simulink model "elec3200lab3"  (R2016a)
settings: Solver=VariableStepAuto  StartTime=0.0  StopTime=10  RelTol=1e-3
settings Model: Creator=古乔  LastModifiedBy=古乔

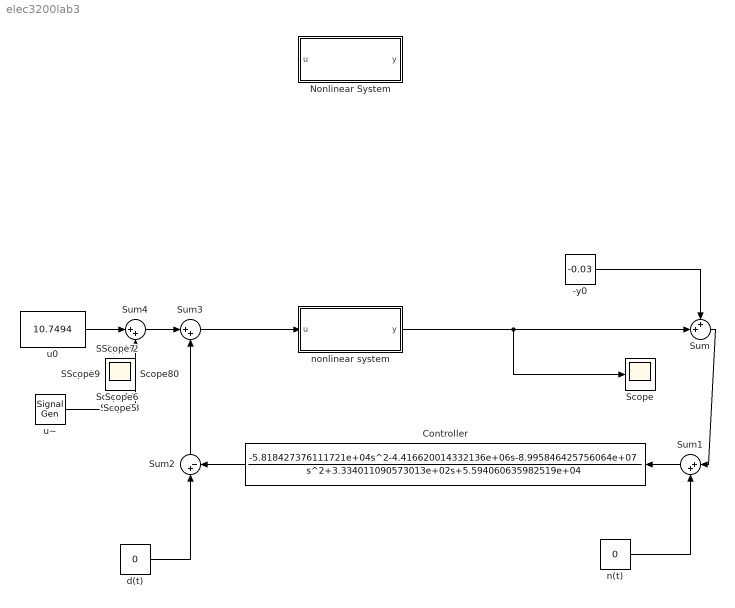
== system elec3200lab3 ==
  -y0 : Constant  Value=-0.03
  Controller : TransferFcn  Numerator=[-5.818427376111721e+04 -4.416620014332136e+06 -8.995846425756064e+07]  Denominator=[1 3.334011090573013e+02 5.594060635982519e+04]
  Nonlinear System : Subsystem
  Scope{,1..14} (15 alike) : Scope
  Sum : Sum  Inputs=++|
  Sum1 : Sum  Inputs=|++
  Sum2 : Sum  Inputs=|+-
  Sum3 : Sum  Inputs=|++
  Sum4 : Sum  Inputs=|++
  "d(t) " : Constant  Value=0
  "n(t) " : Constant  Value=0
  nonlinear system : Subsystem
  u0 : Constant  Value=10.7494
  u~ : SignalGenerator  WaveForm=square  Units=rad/sec
  wires:
  -y0/1 -> Sum/1
  Sum/1 -> Sum1/1
  Sum1/1 -> Controller/1
  "n(t) "/1 -> Sum1/2
  Controller/1 -> Sum2/2
  "d(t) "/1 -> Sum2/1
  Sum2/1 -> Sum3/2
  u0/1 -> Sum4/1
  Sum3/1 -> nonlinear system/1(u)
  nonlinear system/1(y) -> Sum/2, Scope/1
  Sum4/1 -> Sum3/1
  u~/1 -> Sum4/2

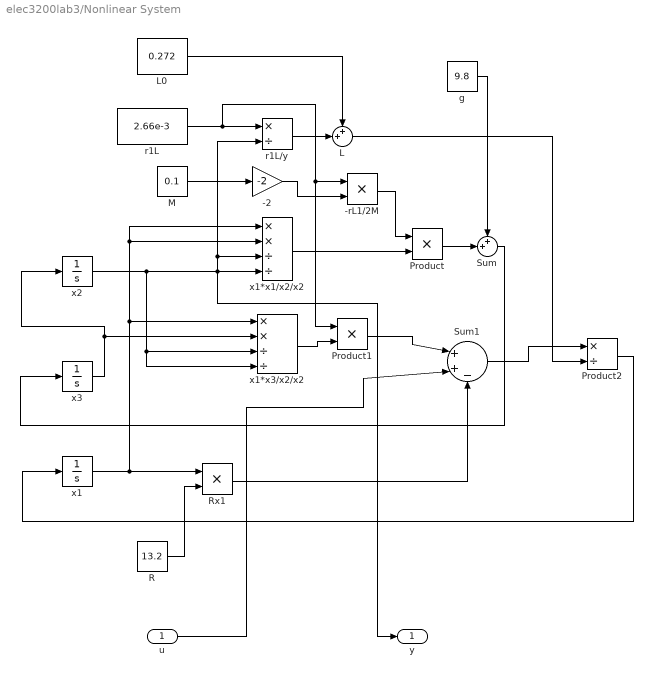
== system elec3200lab3/Nonlinear System ==
  u : Inport
  -2 : Gain  Gain=-2
  -rL1/2M : Product
  L : Sum  Inputs=++|
  L0 : Constant  Value=0.272
  M : Constant  Value=0.1
  Product : Product
  Product1 : Product
  Product2 : Product  Inputs=*/
  R : Constant  Value=13.2
  Rx1 : Product
  Sum : Sum  Inputs=++|
  Sum1 : Sum  Inputs=|++-
  g : Constant  Value=9.8
  r1L : Constant  Value=2.66e-3
  r1L/y : Product  Inputs=*/
  x1 : Integrator  InitialCondition=0.8143
  x1*x1/x2/x2 : Product  Inputs=**//
  x1*x3/x2/x2 : Product  Inputs=**//
  x2 : Integrator  InitialCondition=0.0300
  x3 : Integrator
  y : Outport
  wires:
  x1/1 -> Rx1/1, x1*x1/x2/x2/1, x1*x1/x2/x2/2, x1*x3/x2/x2/1
  x2/1 -> y/1, r1L/y/2, x1*x1/x2/x2/3, x1*x1/x2/x2/4, x1*x3/x2/x2/4, x1*x3/x2/x2/3
  r1L/1 -> Product1/1, -rL1/2M/1, r1L/y/1
  r1L/y/1 -> L/2
  L0/1 -> L/1
  L/1 -> Product2/2
  x3/1 -> x2/1, x1*x3/x2/x2/2
  M/1 -> -2/1
  -2/1 -> -rL1/2M/2
  -rL1/2M/1 -> Product/1
  x1*x1/x2/x2/1 -> Product/2
  Product/1 -> Sum/2
  g/1 -> Sum/1
  Sum/1 -> x3/1
  x1*x3/x2/x2/1 -> Product1/2
  R/1 -> Rx1/2
  u/1 -> Sum1/2
  Product1/1 -> Sum1/1
  Rx1/1 -> Sum1/3
  Sum1/1 -> Product2/1
  Product2/1 -> x1/1

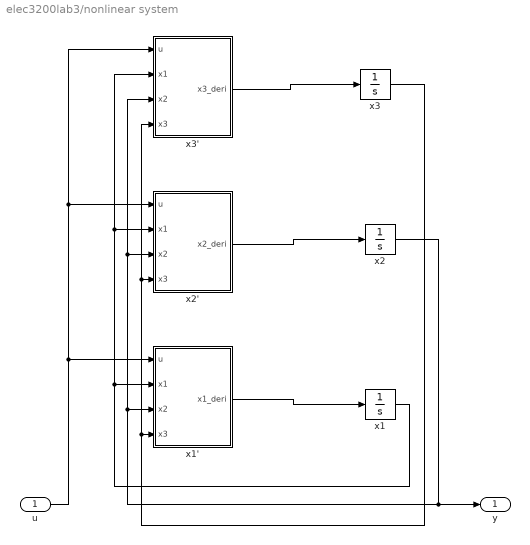
== system elec3200lab3/nonlinear system ==
  u : Inport
  x1 : Integrator  InitialCondition=0.84
  x1' : MATLAB Function  TreatAsAtomicUnit=on
  x2 : Integrator  InitialCondition=0.03
  x2' : MATLAB Function  TreatAsAtomicUnit=on
  x3 : Integrator
  x3' : MATLAB Function  TreatAsAtomicUnit=on
  y : Outport
  wires:
  u/1 -> x3'/1(u), x2'/1(u), x1'/1(u)
  x1'/1(x1_deri) -> x1/1
  x2'/1(x2_deri) -> x2/1
  x3'/1(x3_deri) -> x3/1
  x3/1 -> x3'/4(x3), x2'/4(x3), x1'/4(x3)
  x2/1 -> y/1, x3'/3(x2), x2'/3(x2), x1'/3(x2)
  x1/1 -> x1'/2(x1), x2'/2(x1), x3'/2(x1)

== matlab function elec3200lab3/nonlinear system/x2' ==
  data: u input; x1 input; x2_deri output; x2 input; x3 input
function x2_deri  = cal_dx2(u,x1,x2,x3)
y0 = 0.03;
L0 = 0.272;
R = 13.2;
M = 0.1;
rL1 = 2.66e-3;
g = 9.8;
L = L0 + rL1/x2;

x2_deri = x3;

== matlab function elec3200lab3/nonlinear system/x1' ==
  data: u input; x1 input; x1_deri output; x2 input; x3 input
function x1_deri  = cal_dx1(u,x1,x2,x3)
y0 = 0.03;
L0 = 0.272;
R = 13.2;
M = 0.1;
rL1 = 2.66e-3;
g = 9.8;
L = L0 + rL1/x2;

x1_deri = (u-R*x1+rL1*x1*x3/x2/x2)/L;

== matlab function elec3200lab3/nonlinear system/x3' ==
  data: u input; x1 input; x3_deri output; x2 input; x3 input
function x3_deri  = cal_dx3(u,x1,x2,x3)
y0 = 0.03;
L0 = 0.272;
R = 13.2;
M = 0.1;
rL1 = 2.66e-3;
g = 9.8;
L = L0 + rL1/x2;

x3_deri = -(rL1/2/M)*x1*x1/x2/x2+g;
